simulink library "wt_blockset_v3"  (Simulink 6.0)
settings: Solver=ode45  SolverMode=SingleTasking  StartTime=0.0  StopTime=10.0  RelTol=1e-3
undefined symbols (not defined in the file): f1, get, j, Kmode, Type, u0
libraries: simulink_extras x12, simulink3 x5, simulink x4, dspinverses x1, dspmtrx3 x1, dspsnks4 x1
(part 1 of 7)
Description:
  | Currently the toolbox can run under Release 7.0.0 (Service Pack 1).
  | Since there are major differences between this Matlab Release and the
  | previous ones, it is highly recommended to use the Toolbox just with
  | Release 7.0.0 or higher.
  | 
  | Many thanks for feedbacks and improvements in particular to:
  | - my colleagues from Risø: Anca Hansen, Poul Sørensen, Nic Cutululis
  | - James F. Conroy
  | - Gabrielle Gail
  | 
  | Also, many thanks to all the users.
  | 
  | Florin
settings Model: Creator=Florin iov  LastModifiedBy=fi  ModifiedComment=fi -- Thu Jun 08 10:02:30 2006 -- Version 3.0.19
settings Model: ModifiedHistory=|
  | fi -- Thu Jun 08 10:02:30 2006 -- Version 3.0.19
  | 
  | 
  | fi -- Tue Oct 25 13:03:19 2005 -- Version 3.0.18
  | 
  | 
  | fi -- Tue Oct 25 13:01:51 2005 -- Version 3.0.17
  | 
  | 
  | fi -- Tue Oct 25 13:01:21 2005 -- Version 3.0.16
  | 
  | 
  | fi -- Tue Oct 25 12:57:57 2005 -- Version 3.0.15
  | 
  | 
  | fi -- Tue Oct 25 12:21:51 2005 -- Version 3.0.14
  | 
  | 
  | fi -- Tue Oct 25 12:15:48 2005 -- Version 3.0.13
  | 
  | 
  | fi -- Tue Oct 25 12:00:01 2005 -- Version 3.0.12
  | Updates: Grid Model, Line Model, Wind Model SB, Capacitor Bank Model, Discrete PLL and PI Controller
  | 
  | fi -- Mon Oct 24 09:19:02 2005 -- Version 3.0.11
  | 
  | 
  | fi -- Thu Jun 02 08:52:48 2005 -- Version 3.0.10
  | 
  | 
  | fi -- Thu Jun 02 08:43:54 2005 -- Version 3.0.9
  | 
  | 
  | fi -- Thu Jun 02 08:40:14 2005 -- Version 3.0.8
  | 
  | 
  | fi -- Wed May 25 13:16:38 2005 -- Version 3.0.7
  | 
  | 
  | fi -- Wed May 25 13:08:05 2005 -- Version 3.0.6
  | 
  | 
  | fi -- Wed May 25 11:45:18 2005 -- Version 3.0.5
  | 
  | 
  | fi -- Wed May 25 11:38:20 2005 -- Version 3.0.3
  | 
  | 
  | fi -- Wed May 25 11:38:20 2005 -- Version 3.0.3
  | 
  | 
  | fi -- Wed May 25 11:25:12 2005 -- Version 3.0.2
settings OptimizationCC: BooleanDataType=off
settings DebuggingCC: SolverPrmCheckMsg=none
settings HardwareCC: TargetUnknown=on

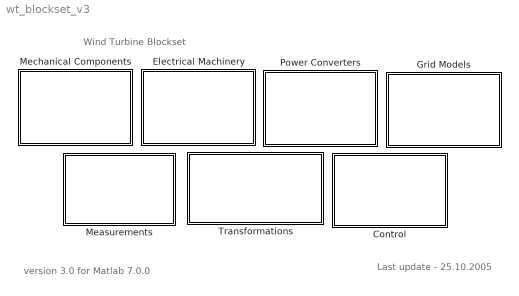
== system wt_blockset_v3 ==
  note: Wind Turbine Blockset
  note: Last update - 25.10.2005
  note: version 3.0 for Matlab 7.0.0
  Control : Subsystem
      mask Display: disp('Control')
  Electrical Machinery : Subsystem
      mask Display: disp('Electrical\nMachinery')
  Grid Models : Subsystem
      mask Display: disp('Grid\nModels')
  Measurements : Subsystem
      mask Display: disp('Measurements')
  Mechanical Components : Subsystem
      mask Display: disp('Mechanical\nComponents')
  Power Converters : Subsystem
      mask Display: disp('Power\nConverters')
  Transformations : Subsystem
      mask Display: disp('Transformations')

== system wt_blockset_v3/Control ==
  note: Control Blocks
  "Active Stall Controller " : Subsystem  mask{K=0.01, Ti=0.0025, ka=500, Kpitch=1000, P=300, avg_wind=11.5, rated_wind=11.8}
      mask prompts: K "Gain Power Controller"; Ti "Integration time constant Power Controller"; ka "Gain anti wind-up Power Controller"; Kpitch "Gain Pitch Controller"; P "Allowed Overpower [kW]"; avg_wind "Average Wind Speed [m/sec]"; rated_wind "Rated Wind Speed"
      mask init:
      | Pallowed=P;
      mask Display: disp('Active\nStall\nController')
  Control P&Q  2 MW DFIG : Subsystem  mask(Control P & Q for double feed induction generator){param=[0.0011, 7e-5, 0.0013, 7.5e-5, 2.9936e-3], p=2, fs=50}
      mask prompts: param "Electrical parameters [Rs Lsgm_s Rr Lsgm_r Lm]"; p "Number of pole pais"; fs "Base frequency [Hz]"
      mask help: Control of active and reactive power in synchronous reference frame for DFIG.
      mask init:
      | Rs=param(1); Lsgm_s=param(2); Rr=param(3); Lsgm_r=param(4);
      | Lm=param(5); Lss=Lsgm_s+Lm; Lrr=Lsgm_r+Lm; D=Lss*Lrr-Lm^2;
      | T=D/Lss; Tpr=(Lm^2)/Lss;
      | tau_1=T/Rr;  tau_2=Rr;
      mask Display: disp('Control\nP&Q')
  PI Controller anti wind-up : Subsystem  mask{K=0.09, Ti=0.016, ka=10, maxim=1000, init_cond=2}
      mask prompts: K "Proportional Constant"; Ti "Integrate constant"; maxim "Limits"; init_cond "initial"
      mask Display: disp('PI')
  WT Controller 2 MW DFIG : Subsystem  mask(Wind Turbine Controller){Kp_power=400, Ti_power=1, Kp_speed=0.02, Ti_speed=10}
      mask prompts: Kp_power "Gain Power Controller"; Ti_power "Integration Time Power Controller"; Kp_speed "Gain Speed Controller"; Ti_speed "Integration Time Speed Controller"
      mask help:
      | Implements the wind turbine controller for a 2MW DFIG WT.
      | Power input is in per unit from the total deliver power.
  control soft starter : Subsystem  TreatAsAtomicUnit=on
      mask Type: Firing angle control for soft starter
      mask Description: Implements the control for soft starter
      mask Display: disp('   ')
  discrete PI Controller anti windup : Subsystem  mask{Kp=2, Ti=0.5, Ka=0, OutLim=1, Ts=1e-2, InitCond=0}
      mask prompts: Kp "Gain"; Ti "Integration Time Constant"; Ka "gain antiwindup"; OutLim "Output limit"; Ts "Sampling time"; InitCond "Initial condition"
      mask Display: disp('Discrete PI')

== system wt_blockset_v3/Electrical Machinery ==
  note: Electrical Machinery Library
  C S-Function based  Models : Subsystem
      mask Display: disp('C S-Function\nbased  Models')
  Simulink Blocks  based Models : Subsystem
      mask Display: disp('Simulink Blocks\n based Models')

== system wt_blockset_v3/Grid Models ==
  note: Sources
  note: Cables & Distribution Lines
  note: others
  note: Transformers
  3-ph line 1 : Subsystem  mask(3-phase distribution line){d=3.3, R=0.115, L=0.19/314, C=0.52e-6}
      mask prompts: d "Line length [km]"; R "Line resistance [ohms/km]"; L "Line inductance [H/km]"; C "Line capacitance [F/km]"
      mask init:
      | Zc=sqrt(L/C);
      | tdelay=d*sqrt(L*C);
      | atten=exp(-(R/2)*d*sqrt(C/L));
      | buffer_size=20000;
  3-ph line 2 : Subsystem  mask(3-phase distribution line){d=4, R=0.115, L=0.2/314, C=0.1e-6}
      mask prompts: d "Line length [km]"; R "Line resistance [ohms/km]"; L "Line inductance [H/km]"; C "Line capacitance [F/km]"
      mask init:
      | Zc=sqrt(L/C);
      | tdelay=d*sqrt(L*C);
      | atten=exp(-(R/2)*d*sqrt(C/L));
      | buffer_size=20000;
  3-phase 3 limb  C S-Function : Subsystem  mask(ABC/abc Dynamic Model of 3-phase 3 limb transformer){power=[2e6 3489], voltage=[31500 690/sqrt(3)], frequency=50, hv_winding=[4.5565 51.227], lv_winding=[2.93 51.227], core_ratio=0.33}
      mask prompts: power "Rated power, No-load losses [Sr (VA), Po (W)]"; voltage "Rated phase voltages [U1r (V), U2r (V)]]"; frequency "Rated frequency [Hz]"; hv_winding "High-voltage windings [Rhv  X_hv] [ohms]"; lv_winding "Low-voltage windings [Rlv X_lv] [ohms]"; core_ratio "Core ratio (l/L)"
      mask help:
      | Implements a dynamic model of a 3-phase 2-windings transformer in natural frame (ABC/abc). Core geometry is taken into account.
      | Connection Type Dyn1.
      mask init:
      | %%%%%%%%%%%%%%%%%%%%%%%%%%%%%%%%%%%%%%%%%%%%%%%%%%%%%%%%%
      | % Coefficients for ABC/abc Model of 3-phase Transformer %
      | %           Core structure is taken into account        %
      | %               Last Update 6.08.2002                   %
      | %%%%%%%%%%%%%%%%%%%%%%%%%%%%%%%%%%%%%%%%%%%%%%%%%%%%%%%%%
      | 
      | %Base power
      | Sbase=power(1);
      | 
      | %No load losses
      | Po=power(2);
      | 
      | %Base HV voltage
      | Ubase_hv=voltage(1);
      | 
      | %Base HV voltage
      | Ubase_lv=voltage(2);
      | 
      | %Base impedance LV
      | Zbase_lv=3*(Ubase_lv^2)/Sbase;
      | 
      | %Transformer turns ratio
      | alpha_T=Ubase_hv/Ubase_lv;
      | 
      | %No load losses per unit
      | Po_pu=Po/Sbase;
      | 
      | %
      | omg=2*pi*frequency;
      | 
      | %High-voltage windings
      | R1=hv_winding(1);
      | X1=hv_winding(2);
      | 
      | %Low-voltage windings
      | R2=lv_winding(1);
      | X2=lv_winding(2);
      | 
      | %%%%%%%%%%%%%%%%%%%%%%%%%%%%%%%%%%%%%%%%%%%%%%%%%%%%%%%%%%%%%
      | 
      | Lsgm=[ X1,     0,     0,     0,     0,     0;...
      |         0,    X1,     0,     0,     0,     0;...
      |         0,     0,    X1,     0,     0,     0;...
      |         0,     0,     0,    X2,     0,     0;...
      |         0,     0,     0,     0,    X2,     0;...
      |         0,     0,     0,     0,     0,    X2]./omg;
      | 
      | 
      | R=[    R1,     0,     0,     0,     0,     0;...
      |         0,    R1,     0,     0,     0,     0;...
      |         0,     0,    R1,     0,     0,     0;...
      |         0,     0,     0,    R2,     0,     0;...
      |         0,     0,     0,     0,    R2,     0;...
      |         0,     0,     0,     0,     0,    R2];
      | 
      | a=core_ratio;
      | 
      | %3limb core
      | %Ideal transformer matrix
      | 
      | k1=-0.5*(1+2*a)/(1+a);
      | k2=-0.5/(1+a);
      | k3=(1+2*a)/(1+a);
      | 
      | Ti=[  1, k1, k2,  1, k1, k2;...
      |      k1, k3, k1, k1, k3, k1;...
      |      k2, k1,  1, k2, k1,  1;...
      |       1, k1, k2,  1, k1, k2;...
      |      k1, k3, k1, k1, k3, k1;...
      |      k2, k1,  1, k2, k1,  1];
      | 
      | T=Ti(1:3,1:3);
      | 
      | dlt=0.001*eye(3,3);
      | 
      | Z=j*(dlt+T);
      | 
      | U=[exp(j*0);exp(-j*2*pi/3);exp(+j*2*pi/3)];
      | 
      | I=Z\U;
      | 
      | Iu=mean(abs(I));
      | 
      | Io_pu=0.002;
      | 
      | PU=real(I'*T*(I));
      | 
      | zeta=Iu/Io_pu;
      | 
      | c=zeta^2*Po_pu/PU;
      | 
      | k=sqrt((zeta^2-c^2)/omg^2);
      | 
      | R0=c*Zbase_lv*alpha_T^2*Ti;
      | L0=k*Zbase_lv*alpha_T^2*Ti;
      | 
      | Re=R+R0;
      | Le=Lsgm+L0;
      | 
      | a=-Le\Re;
      | 
      | b=inv(Le);
      | 
      | init_cond = [0 0 0 0 0 0];
      mask Display: disp('3phase 3 limb\n Transformer')
  3-phase 3 limb  Transformer : Subsystem  mask(ABC/abc Dynamic Model of 3-phase 3 limb transformer){power=[2e6 3489], voltage=[31500 690/sqrt(3)], frequency=50, hv_winding=[4.5565 51.227], lv_winding=[2.93 51.227], core_ratio=0.33}
      mask prompts: power "Rated power, No-load losses [Sr (VA), Po (W)]"; voltage "Rated phase voltages [U1r (V), U2r (V)]]"; frequency "Rated frequency [Hz]"; hv_winding "High-voltage windings [Rhv  X_hv] [ohms]"; lv_winding "Low-voltage windings [Rlv X_lv] [ohms]"; core_ratio "Core ratio (l/L)"
      mask help:
      | Implements a dynamic model of a 3-phase 2-windings transformer in natural frame (ABC/abc). Core geometry is taken into account.
      | Connection Type Dyn1.
      mask init:
      | %%%%%%%%%%%%%%%%%%%%%%%%%%%%%%%%%%%%%%%%%%%%%%%%%%%%%%%%%
      | % Coefficients for ABC/abc Model of 3-phase Transformer %
      | %           Core structure is taken into account        %
      | %               Last Update 6.08.2002                   %
      | %%%%%%%%%%%%%%%%%%%%%%%%%%%%%%%%%%%%%%%%%%%%%%%%%%%%%%%%%
      | 
      | %Base power
      | Sbase=power(1);
      | 
      | %No load losses
      | Po=power(2);
      | 
      | %Base HV voltage
      | Ubase_hv=voltage(1);
      | 
      | %Base HV voltage
      | Ubase_lv=voltage(2);
      | 
      | %Base impedance LV
      | Zbase_lv=3*(Ubase_lv^2)/Sbase;
      | 
      | %Transformer turns ratio
      | alpha_T=Ubase_hv/Ubase_lv;
      | 
      | %No load losses per unit
      | Po_pu=Po/Sbase;
      | 
      | %
      | omg=2*pi*frequency;
      | 
      | %High-voltage windings
      | R1=hv_winding(1);
      | X1=hv_winding(2);
      | 
      | %Low-voltage windings
      | R2=lv_winding(1);
      | X2=lv_winding(2);
      | 
      | %%%%%%%%%%%%%%%%%%%%%%%%%%%%%%%%%%%%%%%%%%%%%%%%%%%%%%%%%%%%%
      | 
      | Lsgm=[ X1,     0,     0,     0,     0,     0;...
      |         0,    X1,     0,     0,     0,     0;...
      |         0,     0,    X1,     0,     0,     0;...
      |         0,     0,     0,    X2,     0,     0;...
      |         0,     0,     0,     0,    X2,     0;...
      |         0,     0,     0,     0,     0,    X2]./omg;
      | 
      | 
      | R=[    R1,     0,     0,     0,     0,     0;...
      |         0,    R1,     0,     0,     0,     0;...
      |         0,     0,    R1,     0,     0,     0;...
      |         0,     0,     0,    R2,     0,     0;...
      |         0,     0,     0,     0,    R2,     0;...
      |         0,     0,     0,     0,     0,    R2];
      | 
      | a=core_ratio;
      | 
      | %3limb core
      | %Ideal transformer matrix
      | 
      | k1=-0.5*(1+2*a)/(1+a);
      | k2=-0.5/(1+a);
      | k3=(1+2*a)/(1+a);
      | 
      | Ti=[  1, k1, k2,  1, k1, k2;...
      |      k1, k3, k1, k1, k3, k1;...
      |      k2, k1,  1, k2, k1,  1;...
      |       1, k1, k2,  1, k1, k2;...
      |      k1, k3, k1, k1, k3, k1;...
      |      k2, k1,  1, k2, k1,  1];
      | 
      | T=Ti(1:3,1:3);
      | 
      | dlt=0.001*eye(3,3);
      | 
      | Z=j*(dlt+T);
      | 
      | U=[exp(j*0);exp(-j*2*pi/3);exp(+j*2*pi/3)];
      | 
      | I=Z\U;
      | 
      | Iu=mean(abs(I));
      | 
      | Io_pu=0.002;
      | 
      | PU=real(I'*T*(I));
      | 
      | zeta=Iu/Io_pu;
      | 
      | c=zeta^2*Po_pu/PU;
      | 
      | k=sqrt((zeta^2-c^2)/omg^2);
      | 
      | R0=c*Zbase_lv*alpha_T^2*Ti;
      | L0=k*Zbase_lv*alpha_T^2*Ti;
      | 
      | Re=R+R0;
      | Le=Lsgm+L0;
      | 
      | a=-Le\Re;
      | 
      | b=inv(Le);
      mask Display: disp('3phase 3 limb\n Transformer')
  3-phase source : Subsystem  mask(3 - Phase Voltage Source){Uf=220, fs=50}
      mask prompts: Uf "Phase voltage [V]"; fs "Fundamental frequency [Hz]"
  Capacitor Bank RC : Subsystem  mask(Capacitor Bank RC){R=1, CmF=21.737}
      mask prompts: R "Series rezistor [ohms]"; CmF "Branch Capacitor [mF]"
      mask init:
      | C=CmF*1e-3;
      mask Display: disp('Capacitor\nBank')
  Capacitor Bank RC modified : Subsystem  mask(Capacitor Bank RC){P=25, Q=500, Vl=0.69}
      mask prompts: P "Dissipated Real Power [W]"; Q "Rated Reactive Power [kVAr]"; Vl "Rated Line Voltage [kV]"
      mask init:
      | Vl = Vl*1e3 ;
      | Q = Q*1e3 ;
      | f = 50 ;
      | omega = 2*pi*f ;
      | 
      | % -------------------------------------------------------------------------
      | 
      | 
      | % Now evaluate the first guess, which is important in Newton-Raphson
      | % algorithms.
      | 
      | % Since the resistance is parasitic in an a real capacitor, R=0 is a decent first guess
      | R = 0 ;
      | % The first guess value for C is the formula for an ideal capacitor
      | C = Q/(Vl^2*omega) ;
      | 
      | % The iterated values for R and C need to be initially at values that are quite different from the first guess values
      | R_prev = 1000 ;
      | C_prev = 1000 ;
      | 
      | % The iteration formula is as follows
      | % -------------------------------------------
      | 
      | %    | a11 a12 |   | dR |     | f(R,C) |
      | %    |         | . |    | = - |        |
      | %    | a21 a22 |   | dC |     | g(R,C) |
      | 
      | %    R(n+1) = R(n) + dR
      | %    C(n+1) = C(n) + dC
      | 
      | %---------------------------------------------
      | 
      | 
      | i = 0 ; % The number of iterations
      | 
      | while((abs(R-R_prev)>0.00000001)|(abs(C-C_prev)>0.00000001))
      |     
      |     R_prev = R ; % Update the previous guess for R
      |     C_prev = C ; % Update the previous guess for C
      |     
      |     % Evaluate the two non-linear functions
      |     f = P*(R^2)+(P/((omega*C)^2))-(Vl^2*R) ;
      |     g = (Q*omega*C*R^2)+(Q/(omega*C))-Vl^2 ;
      | 
      |     % Now get the factors that you require
      |     a11 = P*2*R - Vl^2 ;
      |     a12 = -2*P/(omega^2*C^3) ;
      |     a21 = Q*2*R ;
      |     a22 = (-Q*2/(omega^2*C^3))-(Vl^2/omega^2)-(1/(C^2)) ; 
      | 
      |     A = [a11 a12;a21 a22] ;
      | 
      |     b = [f;g] ;
      | 
      |     y = -(A\b) ; % The MATLAB convention for solving by Gaussian Elimination
      |     
      |     R = R_prev+y(1) ; % Update the guess for R
      |     C = C_prev+y(2) ; % Update the guess for C
      |     
      |     % This loop performs iteration control!!
      |     i = i+1 ;
      |     if i==500000
      |         break ;
      | 	end
      | end
      | R;
      | C;
      mask Display: disp('Capacitor\nBank')
  Capacitor Bank RLC : Subsystem  mask(Capacitor Bank RLC){R=0.0001, X=0.00034, CmF=0.0005}
      mask prompts: R "Series rezistor [ohms]"; X "Reactor [ohms]"; CmF "Capacitance [mF]"
      mask init:
      | L=X/(2*pi*50);
      | C=CmF*1e-3;
      mask Display: disp('Capacitor\nBank')
  Circuit breaker : Subsystem  mask{to=1/50, Ro=100, tc=1/50, Rc=100}
      mask prompts: to "Opening time"; Ro "Opening resistance"; tc "Closing time"; Rc "Closing resistance"
  DC-link circuit : Subsystem  mask(DC-link circuit){R=0.001, CuF=21.737, init_cond=0}
      mask prompts: R "Series rezistor [ohms]"; CuF "Capacitor [uF]"; init_cond "Initial DC-link Voltage [V]"
      mask init:
      | C=CuF*1e-6;
      mask Display: disp('DC\nLink')
  GRID 1 : Subsystem  mask(3 - Phase Voltage Source){Uf=31500, R=0, X=1.5, fs=50}
      mask prompts: Uf "Phase voltage [V]"; R "Resistance"; X "Reactance"; fs "Fundamental frequency [Hz]"
  GRID 2 : Subsystem  mask{fg=50, Vpcc=30000, Ssc=20, phi_grid=80, Rf=0.31, SCR=5, tsc=0.3, td=0.5}
      mask prompts: fg "fgrid [Hz]"; Vpcc "Vpcc line-line  rms [V]"; Ssc "Short-circuit Power (MVA)"; phi_grid "Grid angle [degrees]"; Rf "Short-circuit resistance"; SCR "Short-circuit ratio x/r"; tsc "Short-circuit occurance"; td "Short-circuit duration"
      mask init:
      | V1=Vpcc/sqrt(3);
      | 
      | tg_alpha=tan(phi_grid*pi/180);
      | Zsc=Vpcc^2/(Ssc*1e6);
      | 
      | R=sqrt(Zsc^2/(1+tg_alpha^2));
      | X=R*tg_alpha;
      | L=X/(2*pi*50);
      | 
      | %Short-circuit inductance
      | Lf=SCR*Rf/(2*pi*50);
  Harmonic Voltage Source : Subsystem  mask(Harmonic Voltage Source){phase_o=178.2, h3=on, h5=on, h7=on, h9=on, h11=on, h13=on}
      mask prompts: phase_o "Initial phase [deg]"; h3 "Insertion of 3rd harmonic"; h5 "Insertion of 5th harmonic"; h7 "Insertion of 7th harmonic"; h9 "Insertion of 9th harmonic"; h11 "Insertion of 11th harmonic"; h13 "Insertion of 13th harmonic"
      mask help: Implements a harmonic voltage source according with Standard EN61000-2-2.
      mask init:
      | gama_0=phase_o*pi/180;
  Voltage  source complex : Subsystem  mask(3 - Phase Voltage Source){Uf=960}
      mask prompts: Uf "Phase voltage [V]"

== system wt_blockset_v3/Measurements ==
  note: Measurements
  Discrete PLL : Subsystem  mask(Discrete PLL){Kp=92, Ti=0.1739, Ka=10, limit=500, Vrms=230, fgrid=50, ffilter=10, Ts=1/5000, init_cond=[0 0 0 230]}
      mask prompts: Kp "Gain Controller"; Ti "Integration Time Controller"; Ka "Gain Antiwindup Controller"; limit "Limit Output Controller"; Vrms "RMS Voltage"; fgrid "Fundamental frequency"; ffilter "Filter cut-off frequency"; Ts "Sampling Time"; init_cond "Initial Condition Integrators"
      mask help: implements a discrete Phase Locked Loop.
      mask Display: disp('Discrete PLL')
  Moving Average Filter : Subsystem  mask(Moving Average Filter){Tav=60, init=10}
      mask prompts: Tav "Averaging time interval [sec]"; init "Initial condition"
      mask help: Implements a Moving average filter in time domain
      mask Display: disp('Moving\nAverage')
  P & Q dq : Subsystem
      mask Type: P & Q 1st approach
      mask Description: Calculate active and reactive power based on dq components
      mask Display: disp('P&Q')
  P & Q mono phase : Subsystem  mask(Active & Reactive Power ){f=50}
      mask prompts: f "Fundamental frequency (Hz):"
      mask Display: disp('P&Q\n 1 phase')
  P & Q three phase : Subsystem  mask(Active & Reactive Power ){f=50}
      mask prompts: f "Fundamental frequency (Hz):"
      mask Display: disp('P&Q\n 3-phase')
  Period : Subsystem
      mask Type: Period calculator
      mask Description: Find period for a sinusoidal signals.
      mask Display: disp('')
  Phase Locked Loop : Subsystem  mask(Phase Locked Loop){fs=50, Kp=180.03, Ti=0.00786}
      mask prompts: fs "Fundamental frequency (Hz):"; Kp "Proportional coefficient"; Ti "Integration time constant [sec]"
      mask help: Implements a Phase Locked Loop for grid angle detection
      mask Display: disp('PLL')
  S complex : Subsystem
      mask Type: P & Q
      mask Description: Calculate active and reactive power based on complex inputs
      mask Display: disp('S')
  average wind : Subsystem  mask(Computes the average value of the wind on a given interval){T_period=60, T_sample=0.05}
      mask prompts: T_period "Time period [sec]"; T_sample "Sample time [sec]"
      mask init:
      | N_samples=T_period/T_sample;
      mask Display: disp('Average\nwind')
  power spectra : Subsystem  mask(power spectra){t_sample=0.05}
      mask prompts: t_sample "Sample period"

== system wt_blockset_v3/Mechanical Components ==
  note: Wind Models
  note: Gearbox Models
  note: Rotor Models
  One-mass model : Subsystem  mask{J=90}
      mask prompts: J "Moment of inertia [Nm2]"
      mask Display: disp('E M')
  One-mass model with gear-box : Subsystem  mask(Simple Gearbox){Jem=90, Jwt=49.5e5, K=83.531, init_speed=1.87355}
      mask prompts: Jem "Electric machinery - Moment of inertia [kg m2]"; Jwt "Wind turbine rotor - Moment of inertia [kg*m2]"; K "Gearbox ratio"; init_speed "Initial condition [omg_wt (rad/sec)]"
      mask init:
      | J=Jem*K^2+Jwt;
      mask Display: disp('E M\nGear box')
  Two-mass model : Subsystem  TreatAsAtomicUnit=on  mask(Gearbox with torsional torque){Jem=90, Jwt=49.5e5, Kshaft=114e6, Dshaft=755.658e3, Kgear=83.531, init=[156.5 1.87355]}
      mask prompts: Jem "Electric machine - Moment of inertia:  Jem [ kg*m2]"; Jwt "Wind turbine rotor - Moment of inertia:  Jwt [kg*m2]"; Kshaft "Shaft stiffness:  Kshaft [ Nm/rad]"; Dshaft "Damping coeficient of shaft:  Dshaft [Nm sec/rad]"; Kgear "Gearbox ratio"; init "Initial conditions [omg_em (rad/sec), omg_wt (rad/sec) ]"
      mask help: Implements a gearbox with torsional torque.
      mask Display: disp('Drive Train')
  Two-mass model 'C' S-Function : Subsystem  TreatAsAtomicUnit=on  mask(Gear box with torsional torques){Jem=90, Jwt=49.5e5, Kshaft=114e6, Dshaft=755.658e3, Kgear=83.531, init_cond=[156.5 0 1.87355 0]}
      mask prompts: Jem "Electric machine - Moment of inertia:  Jem [ kg*m2]"; Jwt "Wind turbine rotor - Moment of inertia:  Jwt [kg*m2]"; Kshaft "Shaft stiffness:  Kshaft [ Nm/rad]"; Dshaft "Damping coeficient of shaft:  Dshaft [Nm sec/rad]"; Kgear "Gearbox ratio"; init_cond "Initial conditions [omg_em(rad/s) th_em(rad) omg_wtr(rad/s) th_wtr(rad)]"
      mask help:
      | Implemets the dynamic model of a gearbox with torsional torques.
      | Equations are written at the low speed shaft (wind turbine side).
      mask Display: disp('Drive Train')
  Wind Model SB-1 : Subsystem  TreatAsAtomicUnit=on  mask(Wind Model using Simulink Band-limited white noise generator){D_rotor=72, v_mean=10, roughness=600, turb_int=12, T_sample=0.05}
      mask prompts: D_rotor "Rotor diameter [m]"; v_mean "Average wind speed [m/sec]"; roughness "Length scale [m]"; turb_int "Turbulence intensity [%]"; T_sample "Sample time [sec]"
      mask help:
      | Implements a rotor wind model developped by RISOE National Laboratory based on Kaimal spectra. The model takes into account the rotational turbulences and the tower shadow.
      | This model uses the built-in band-limited white noise generator from Simulink with different seeds.
      mask init:
      | r = D_rotor/2;
      | sigma = v_mean*turb_int/100;
      | var = sigma^2;
      | c = roughness/(2*pi*v_mean);
      | d = r/v_mean;
      | trans=sigma*sqrt(roughness/v_mean);
      | random=[256, 894, 31];
      mask Display: disp('Wind\nModel\n(SB-1)')
  Wind Model SB-2 : Subsystem  TreatAsAtomicUnit=on  mask(Wind Model using Simulink Band-limited white noise generator){D_rotor=72, L=600, turb_int=12, T_sample=0.05}
      mask prompts: D_rotor "Rotor diameter [m]"; L "Length scale [m]"; turb_int "Turbulence intensity [%]"; T_sample "Sample time [sec]"
      mask help:
      | Implements a rotor wind model developped by RISOE National Laboratory based on Kaimal spectra. The model takes into account the rotational turbulences and the tower shadow.
      | This model uses the built-in band-limited white noise generator from Simulink
      mask init:
      | r = D_rotor/2;
      | random=[256, 894, 31];
      mask Display: disp('Wind\nModel\n(SB-2)')
  Wind Model ZA-1 : Subsystem  TreatAsAtomicUnit=on  mask(Wind Model using Marsaglia's Ziggurat Algorithm){D_rotor=72, v_mean=10, roughness=600, turb_int=12, T_sample=0.05}
      mask prompts: D_rotor "Rotor diameter [m]"; v_mean "Average wind speed [m/sec]"; roughness "Length scale [m]"; turb_int "Turbulence intensity [%]"; T_sample "Sample time [sec]"
      mask help:
      | Implements a rotor wind model developped by RISOE National Laboratory based on Kaimal spectra. The model takes into account the rotational turbulences and the tower shadow.
      | The white noise generators uses a new block based on a 'C' S-Function which implements the Marsaglia's Ziggurat Algorithm.
      mask init:
      | r = D_rotor/2;
      | sigma = v_mean*turb_int/100;
      | var = sigma^2;
      | c = roughness/(2*pi*v_mean);
      | d = r/v_mean;
      | trans=sigma*sqrt(roughness/v_mean);
      mask Display: disp('Wind\nModel\n(ZA-1)')
  Wind Model ZA-2 : Subsystem  TreatAsAtomicUnit=on  mask(Wind Model using Marsaglia's Ziggurat Algorithm){D_rotor=72, L=600, turb_int=12, T_sample=0.05}
      mask prompts: D_rotor "Rotor diameter [m]"; L "Length scale [m]"; turb_int "Turbulence intensity [%]"; T_sample "Sample time [sec]"
      mask help:
      | Implements a rotor wind model developped by RISOE National Laboratory based on Kaimal spectra. The model takes into account the rotational turbulences and the tower shadow.
      | The white noise generators uses a new block based on a 'C' S-Function which implements the Marsaglia's Ziggurat Algorithm.
      mask init:
      | r = D_rotor/2;
      mask Display: disp('Wind\nModel\n(ZA-2)')
  Wind Turbine Rotor Active Stall : Subsystem  mask(Aerodynamic model for wind turbine){R=40, ro_air=1.25, cut_in=3, cut_out=25, Tact=0}
      mask prompts: R "Blade radius [m]"; ro_air "Air density [kg m3]"; cut_in "Cut in speed [m/sec]"; cut_out "Cut out speed [m/sec]"; Tact "Time constant for pitch actuator [sec]"
      mask init:
      | load cp_cq;
      | Ctorque=cq(2:5:102,2:5:182);
      | clear Cp cq
      mask Display: plot(20,0,120,200,[45,35,35,45,75,75,45],[85,92,108,115,115,85,85],[55,50,70,65],[115,180,190,115],[55,50,70,65],[85,10,20,85],[75,85],[102,102],[75,85],[98,98],[105,85,85,105],[80,85,115,120])
  Wind Turbine Rotor Variable Pitch : Subsystem  mask(Aerodynamic model for wind turbine){R=40, ro_air=1.25, cut_in=3, cut_out=25, Tact=0}
      mask prompts: R "Blade radius [m]"; ro_air "Air density [kg m3]"; cut_in "Cut in speed [m/sec]"; cut_out "Cut out speed [m/sec]"; Tact "Time constant for pitch actuator [sec]"
      mask init:
      | load cp_cq;
      | Ctorque=cq(2:5:102,2:5:182);
      | clear Cp cq
      mask Display: plot(20,0,120,200,[45,35,35,45,75,75,45],[85,92,108,115,115,85,85],[55,50,70,65],[115,180,190,115],[55,50,70,65],[85,10,20,85],[75,85],[102,102],[75,85],[98,98],[105,85,85,105],[80,85,115,120])

== system wt_blockset_v3/Power Converters ==
  note: Power Converters Models
  note: Power Converters RMS Models
  note: Modulation Strategies
  3-phase Diode Bridge Rectifier : Subsystem
      mask Type: 3 phase Diode Bridge Rectifier
      mask Description: Implements a model for 3 phase Diode Bridge Rectifier.
      mask Display: disp('')
  Average PWM Strategy : Subsystem  mask(Average sinusoidal PWM Strategy with Simulink Blocks){third=on}
      mask prompts: third "Insertion of third harmonic"
      mask help: Implements an average model of a sinusoidal PWM strategy using Simulink Blocks.
      mask Display: disp('Average\nPWM')
  Average SVM Strategy : Subsystem
      mask Type: Average SVM Strategy with Simulink Blocks
      mask Description: Implements an average model of a SV-PWM strategy using Simulink Blocks.
      mask Display: disp('Average\nSVM')
  Average SVM Strategy C_Sfun : Subsystem
      mask Type: Average SVM Strategy C-SFun
      mask Description: Implements an average model of a SV-PWM strategy using a C-SFunction.
      mask Display: disp('Average\nSVM')
  RMS - Soft Starter : Subsystem  mask(RMS Model for Soft Starter){}
      mask help: Implements an RMS model for soft-starter based on a look-up table for extincton angle of the SCR.
      mask init:
      | ext_angle_ss%%%%%%%%%%%%%%%%%%%%%%%%%%%%%%%%%%%%%%%%%%%
      | % Extinction angle tabel for Soft Starter %
      | %       Last Update 10.05.2002            %
      | %%%%%%%%%%%%%%%%%%%%%%%%%%%%%%%%%%%%%%%%%%%
      | 
      | ext_angle=[ 180  180   180  180   180   180   180   180   180   180   180   180   180;...
      |             195  195   195  195   195   195   194.9 194.8 194.6 193.9 192.4 189   180;...
      |             210  210   210  209.9 209.7 209.3 208.6 207.5 205.7 202.9 198.5 191.5 180;...
      |             225  225   225  225   224.2 222.8 220.9 218.1 214.3 209.1 202.1 192.8 180;...
      |             240  240   240  240   240   237.1 233.2 228.2 221.9 214.2 204.9 193.6 180;...
      |             255  255   255  255   255   255   247.9 239.5 230   219.3 207.4 194.3 180;...
      |             270  270   270  270   270   270   270   255   240   225   210   195   180];
  SVM Strategy : Subsystem  mask(SVM-Strategy){fs=1000, Udc=600, td=3.2e-6, mpw=5.6e-6, mct=.4e-6*10, dp=0}
      mask prompts: fs "Parameters:Switching sampling frequency 'fs' [Hz] :"; Udc "DC Link voltage 'Udc' [V] :"; td "Inverter Deadtime 'td' [sec] :"; mpw "Minimum Puls-Width 'mpw' [sec] :"; mct "CPU cycle time 'cmt' [sec] :"; dp "Pulse-Dropping : 0-disabled, 1-enabled"
      mask help: SPACE VECTOR MODULATION - based PWM VSC
      mask Display: plot(0,0,100,100,[3,5,5,10,10,15,15,25,25,30,30,40,40,45,45,50,50,55,55,60,60,70,70,75,75,85,85,90,90,95,95,97],[50,50,10,10,50,50,10,10,50,50,10,10,50,50,10,10,90,90,50,50,90,90,50,50,90,90,50,50,90,90,50,50],[2,98],[50,50])
  Sinus PWM : Subsystem  mask(Sinus PWM Strategy){mf=15, f1=50}
      mask prompts: mf "Amplitude modulation index"; f1 "Fundamental frequency"
  Soft-Starter : Subsystem  mask(Soft Starter){ConType=Delta, fs=50, init=[0 1 1]}
      mask prompts: ConType "Connection Type"; fs "Fundamental frequency [Hz]"; init "Initial states"
      mask help: Implements a Soft-Starter model for star, delta and branch-delta connection using switching functions.
      mask init:
      | init_a=init(1);
      | init_b=init(2);
      | init_c=init(3);
      mask StyleString: popup(Star|Delta|Branch Delta),edit,edit
  Switching PWM Strategy : Subsystem  mask(Switching sinusoidal PWM with Simulink Blocks){carrier=1000, dead_time=3.2e-6, min_pw=5e-6, dp=on, third=on}
      mask prompts: carrier "Carrier frequency [Hz]"; dead_time "Dead time [sec]"; min_pw "Minimum pulse width [sec]"; dp "Pulse dropping"; third "Insertion of third harmonic"
      mask help: Implements a switching model of a sinusoidal PWM strategy using Simulink Blocks.
      mask init:
      | mpw=0.5*min_pw;
      mask Display: disp('Switching\nPWM')
  Switching SVM Strategy : Subsystem  mask(Switching SVM Strategy with Simulink Blocks){fsw=4000, dead_time=3.2e-6, min_pw=5e-6, dp=off}
      mask prompts: fsw "Switching frequency"; dead_time "Dead time [sec]"; min_pw "Minimum pulse width [sec]"; dp "Pulse dropping"
      mask help: Implements a switching model of a SV-PWM strategy using Simulink Blocks.
      mask init:
      | Tsw=1/fsw;
      | mpw=0.5*min_pw;
      mask Display: disp('Switching\nSVM')
  Switching SVM Strategy C_Sfun : Subsystem  mask(Switching SVM Strategy){fsw=4000, dead_time=3e-6, min_pw=5e-6, dp=off}
      mask prompts: fsw "Switching frequency [Hz]"; dead_time "Dead time [sec]"; min_pw "Minimum pulse width [sec]"; dp "Puls dropping"
      mask help: Implements a switching model for SV-PWM using C-SFunction
      mask init:
      | Tsw=1/fsw;
      | mpw=0.5*min_pw;
      mask Display: disp('Switching\nSVM\nC-SFun')
  Voltage Source Converter : Subsystem
      mask Type: Voltage Source Converter - star connected loads
      mask Description:
      | Implements a Voltage Source Converter (Rectifier or Inverter)
      | using switching functions.
      | - input S_ABC is          discret (0,1) => switching model.
      | - input S_ABC is continuous (0...1) =>   average model.
      mask Display: disp('VSC')

== system wt_blockset_v3/Transformations ==
  note: Transformations
  ABC->Mag&Phase : Subsystem
      mask Type: RMS&phase calculator
      mask Description: Calculate the RMS value and phase angle for a 3 phase input.
      mask Display: disp('')
  "DQ -> Complex" : Subsystem
      mask Type: DQ -> Complex
      mask Description: Transformation of dq variables into complex form
  "abc -> dq0" : Subsystem
      mask Description: Implements  ABC -> DQ  transformation
  "dq0 -> abc" : Subsystem
      mask Type: DQ -> ABC
      mask Description: Implements DQ -> ABC transformation
      mask Display: disp(' ')
  "phase -> line currents" : Subsystem
      mask Type: Transformation phase to line currents
      mask Description: Transformation of phase currents into line currents
      mask Display: disp('')
  phase->line voltages : Subsystem
      mask Type: Transformation phase to line voltages
      mask Description: Transformation of phase currents into line voltages
      mask Display: disp('')

== system wt_blockset_v3/Control/Active Stall Controller  ==
  wind : Inport  Port=1  LatchInput=off
  Ps : Inport  Port=2  LatchInput=off
  Pm : Inport  Port=3  LatchInput=off
  Enable : EnablePort  StatesWhenEnabling=reset
  Data Type Conversion : DataTypeConversion  SaturateOnIntegerOverflow=on  RndMeth=Zero
  Gain1 : Gain  Gain=1e-3  SaturateOnIntegerOverflow=on
  Gain2 : Gain  Gain=1*1e-3  SaturateOnIntegerOverflow=on
  MAF_wind : Subsystem  mask(Moving Average Filter){Tav=60, init=11.5}
      mask prompts: Tav "Averaging time interval [sec]"; init "Initial condition"
      mask help: Implements a Moving average filter in time domain
      mask Display: disp('Moving\nAverage')
  MAF_wind1 : Subsystem  mask(Moving Average Filter){Tav=5, init=1.8e6}
      mask prompts: Tav "Averaging time interval [sec]"; init "Initial condition"
      mask help: Implements a Moving average filter in time domain
      mask Display: disp('Moving\nAverage')
  Pitch System : Subsystem
  Power Controller : Subsystem
  Sample and Hold : Subsystem  TreatAsAtomicUnit=on  mask(Sample and Hold){trig=Rising edge, initCond=-1}
      mask prompts: trig "Trigger type:"; initCond "Initial condition:"
      mask help: Sample and hold input signal.
      mask init:
      | switch trig
      | case 1, s='rising';
      | case 2, s='falling';
      | case 3, s='either';
      | end
      | set_param([gcb '/Trigger'],'triggertype',s);
      mask Help: web(dspbhelp);
      mask StyleString: popup(Rising edge|Falling edge|Either edge),edit
      mask Display: disp('S/H')
  Saturation2 : Saturate  UpperLimit=-2  LowerLimit=-25
  Sum : Sum  Inputs=|+-  SaturateOnIntegerOverflow=on
  Switch : Switch  Threshold=0.5  SaturateOnIntegerOverflow=on
  control : Subsystem
  meas5 : Constant  Value=-Pallowed
  overpower  detection4 : RelationalOperator  Operator=>
  theta : Fcn  Expr=0.00068942619218*u(1)^3-0.04716431372377*u(1)^2+0.03911165958433*u(1)+2.45265812747683
  trigger : Subsystem
  pitch : Outport  InitialOutput=[-2.5]
  wires:
  Sum/1 -> overpower  detection4/2, Power Controller/1(error)  "error"
  Switch/1 -> Sample and Hold/1(In)
  Power Controller/1(pitch) -> Switch/3
  theta/1 -> Saturation2/1
  MAF_wind/1(Out) -> theta/1, control/1(av_wind)
  Pitch System/1(Out) -> pitch/1
  wind/1 -> MAF_wind/1(In)
  Ps/1 -> Gain1/1
  Pm/1 -> MAF_wind1/1(In)
  trigger/1(trigger) -> Sample and Hold/Trigger
  meas5/1 -> overpower  detection4/1
  overpower  detection4/1 -> Data Type Conversion/1
  Data Type Conversion/1 -> trigger/1(overpower)  "overpower"
  Saturation2/1 -> Switch/1  "optimum pitch"
  Sample and Hold/1(" ") -> Pitch System/1(In), Power Controller/2(aw)
  control/1(cs) -> Switch/2
  Gain1/1 -> Sum/1
  Gain2/1 -> Sum/2, control/2(error)
  MAF_wind1/1(Out) -> Gain2/1

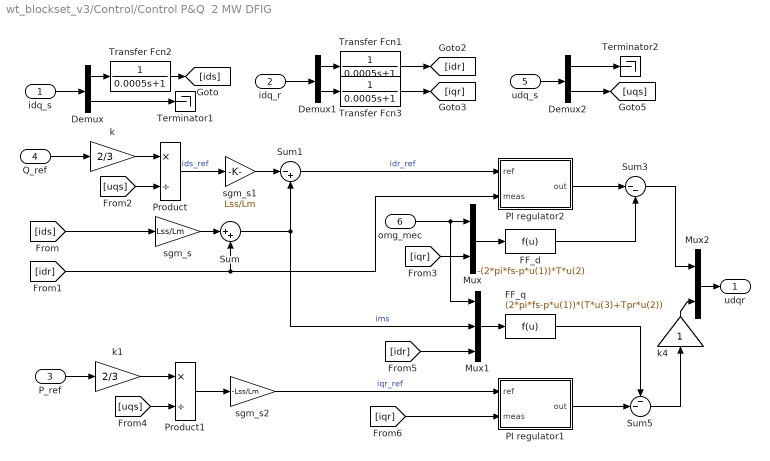
== system wt_blockset_v3/Control/Control P&Q  2 MW DFIG ==
  idq_s : Inport  Port=1  LatchInput=off
  idq_r : Inport  Port=2  LatchInput=off
  P_ref : Inport  Port=3  LatchInput=off
  Q_ref : Inport  Port=4  LatchInput=off
  udq_s : Inport  Port=5  LatchInput=off
  omg_mec : Inport  Port=6  LatchInput=off
  Demux : Demux  Outputs=2
  Demux1 : Demux  Outputs=2
  Demux2 : Demux  Outputs=2
  FF_d : Fcn  Expr=-(2*pi*fs-p*u(1))*T*u(2)
  FF_q : Fcn  Expr=(2*pi*fs-p*u(1))*(T*u(3)+Tpr*u(2))
  Mux : Mux  Inputs=2
  Mux1 : Mux  Inputs=3
  Mux2 : Mux  Inputs=2
  PI regulator1 : Subsystem  mask{K=0.002, Ti=0.04, ka=10, maxim=400, init_cond=0}
      mask prompts: K "Proportional Constant"; Ti "Integrate constant"; maxim "Limits"; init_cond "initial"
  PI regulator2 : Subsystem  mask{K=0.003, Ti=0.04, ka=10, maxim=400, init_cond=0}
      mask prompts: K "Proportional Constant"; Ti "Integrate constant"; maxim "Limits"; init_cond "initial"
  Product : Product  Inputs=*/  SaturateOnIntegerOverflow=on  InputSameDT=on
  Product1 : Product  Inputs=*/  SaturateOnIntegerOverflow=on  InputSameDT=on
  Sum : Sum  Inputs=|++  SaturateOnIntegerOverflow=on  InputSameDT=on
  Sum1 : Sum  Inputs=|-+  SaturateOnIntegerOverflow=on  InputSameDT=on
  Sum3 : Sum  Inputs=|--  SaturateOnIntegerOverflow=on  InputSameDT=on
  Sum5 : Sum  Inputs=--|  SaturateOnIntegerOverflow=on  InputSameDT=on
  Terminator1 : Terminator
  Terminator2 : Terminator
  Transfer Fcn1 : TransferFcn  Denominator=[0.0005 1]
  Transfer Fcn2 : TransferFcn  Denominator=[0.0005 1]
  Transfer Fcn3 : TransferFcn  Denominator=[0.0005 1]
  k : Gain  Gain=2/3  SaturateOnIntegerOverflow=on
  k1 : Gain  Gain=2/3  SaturateOnIntegerOverflow=on
  k4 : Gain  Orientation=up  SaturateOnIntegerOverflow=on
  sgm_s : Gain  Gain=Lss/Lm  SaturateOnIntegerOverflow=on
  sgm_s1 : Gain  Gain=Lss/Lm  SaturateOnIntegerOverflow=on
  sgm_s2 : Gain  Gain=-Lss/Lm  SaturateOnIntegerOverflow=on
  udqr : Outport
  wires:
  idq_s/1 -> Demux/1
  idq_r/1 -> Demux1/1
  Demux/1 -> Transfer Fcn2/1
  Demux/2 -> Terminator1/1
  Demux1/2 -> Transfer Fcn3/1
  [ids] -> sgm_s/1
  sgm_s/1 -> Sum/1
  [idr] -> Sum/2, PI regulator2/2(meas)
  udq_s/1 -> Demux2/1
  Demux2/1 -> Terminator2/1
  Demux2/2 -> [uqs]
  Q_ref/1 -> k/1
  k/1 -> Product/1
  [uqs] -> Product/2
  Product/1 -> sgm_s1/1  "ids_ref"
  Sum/1 -> Sum1/2, Mux1/2  "ims"
  PI regulator2/1(out) -> Sum3/1
  omg_mec/1 -> Mux/1, Mux1/1
  Mux/1 -> FF_d/1
  [iqr] -> Mux/2
  Sum3/1 -> Mux2/1
  P_ref/1 -> k1/1
  k1/1 -> Product1/1
  [uqs] -> Product1/2
  Product1/1 -> sgm_s2/1
  sgm_s2/1 -> PI regulator1/1(ref)  "iqr_ref"
  Mux1/1 -> FF_q/1
  PI regulator1/1(out) -> Sum5/2
  [idr] -> Mux1/3
  Sum5/1 -> k4/1
  Mux2/1 -> udqr/1
  sgm_s1/1 -> Sum1/1
  Sum1/1 -> PI regulator2/1(ref)  "idr_ref"
  FF_d/1 -> Sum3/2
  [iqr] -> PI regulator1/2(meas)
  Demux1/1 -> Transfer Fcn1/1
  Transfer Fcn2/1 -> [ids]
  Transfer Fcn1/1 -> [idr]
  Transfer Fcn3/1 -> [iqr]
  k4/1 -> Mux2/2
  FF_q/1 -> Sum5/1

== system wt_blockset_v3/Control/PI Controller anti wind-up ==
  error : Inport  Port=1  LatchInput=off
  1/T : Gain  Gain=1/Ti  SaturateOnIntegerOverflow=on
  Integrator : Integrator  InitialCondition=init_cond
  P1 : Gain  Gain=K  SaturateOnIntegerOverflow=on
  P2 : Gain  Orientation=left  Gain=ka  SaturateOnIntegerOverflow=on
  Saturation : Saturate  UpperLimit=maxim  LowerLimit=-maxim
  Sum1 : Sum  Inputs=|+-  SaturateOnIntegerOverflow=on  InputSameDT=on
  Sum2 : Sum  Inputs=++|  SaturateOnIntegerOverflow=on  InputSameDT=on
  Sum4 : Sum  Orientation=left  Inputs=+-|  SaturateOnIntegerOverflow=on  InputSameDT=on
  out : Outport  InitialOutput=0
  wires:
  Sum1/1 -> 1/T/1
  Integrator/1 -> Sum2/2
  1/T/1 -> Integrator/1
  error/1 -> P1/1
  P1/1 -> Sum1/1, Sum2/1
  P2/1 -> Sum1/2
  Sum2/1 -> Sum4/1, Saturation/1
  Sum4/1 -> P2/1
  Saturation/1 -> out/1, Sum4/2

== system wt_blockset_v3/Control/WT Controller 2 MW DFIG ==
  Pref_pu : Inport  Port=1  LatchInput=off
  Pmeas_pu : Inport  Port=2  LatchInput=off
  omg_meas : Inport  Port=3  LatchInput=off
  AAL : TransferFcn  Orientation=left  Denominator=[1e-4 1]
  Gain Scheduling : S-Function  Orientation=left  FunctionName=sfun_polyval  Parameters=coefs  mask(Polyval){coefs=[-2.0919e-008, 2.0362e-006, -8.1788e-005 1.7529e-003, -2.1671e-002, 1.5651e-001, -6.4415e-001, 1.4533e+000]}
      mask prompts: coefs "Polynomial coefficients:"
      mask help: Polynomial evaluation. Calculates P(u) given by the polynomial coefficient array P. P is sorted highest order to lowest order, the form accepted by MATLAB's polyval function.
      mask init:
      | if isempty(coefs)
      |   str = 'O(P) = ???';
      | else
      |   str = sprintf('O(P) = %d',length(coefs)-1);
      | end
      mask Display:
      | text(0.5,0.75, 'P(u)','horizontalAlignment','center')
      | text(0.5,0.25, str,'horizontalAlignment','center')
  Limit Power : Saturate  UpperLimit=0.6272  LowerLimit=0.0672
  Limit speed range : Saturate  UpperLimit=175.679  LowerLimit=83.77
  Optimum  speed : S-Function  FunctionName=sfun_polyval  Parameters=coefs  mask(Polyval){coefs=[-890.33 1543.7 -1074.6 467.9 53.548]}
      mask prompts: coefs "Polynomial coefficients:"
      mask help: Polynomial evaluation. Calculates P(u) given by the polynomial coefficient array P. P is sorted highest order to lowest order, the form accepted by MATLAB's polyval function.
      mask init:
      | if isempty(coefs)
      |   str = 'O(P) = ???';
      | else
      |   str = sprintf('O(P) = %d',length(coefs)-1);
      | end
      mask Display:
      | text(0.5,0.75, 'P(u)','horizontalAlignment','center')
      | text(0.5,0.25, str,'horizontalAlignment','center')
  Pitch System : Subsystem
  Power Controller : Subsystem  mask{K=Kp_power, Ti=Ti_power, ka=10, maxim=1, init_cond=0}
      mask prompts: K "Proportional Constant"; Ti "Integrate constant"; maxim "Limits"; init_cond "initial"
  Speed Controller : Subsystem  mask{K=Kp_speed, Ti=Ti_speed, ka=10, maxim=1000, init_cond=1}
      mask prompts: K "Proportional Constant"; Ti "Integrate constant"; maxim "Limits"; init_cond "initial"
  pitch : Outport
  Pref : Outport  Port=2
  wires:
  AAL/1 -> Gain Scheduling/1
  Gain Scheduling/1 -> Power Controller/3(Gain)
  Pref_pu/1 -> Power Controller/1(Ref), Limit Power/1
  Pmeas_pu/1 -> Power Controller/2(Meas)
  Power Controller/1(Out) -> Pitch System/1(In)
  Limit Power/1 -> Optimum  speed/1
  Optimum  speed/1 -> Limit speed range/1
  Limit speed range/1 -> Speed Controller/1(ref)
  Speed Controller/1(out) -> Pref/1
  omg_meas/1 -> Speed Controller/2(meas)
  Pitch System/1(Out) -> pitch/1, AAL/1

== system wt_blockset_v3/Control/control soft starter ==
  Enable : EnablePort
  Constant : Constant
  Constant1 : Constant  Value=110
  Gain1 : Gain  Gain=150  SaturateOnIntegerOverflow=on
  Integrator : Integrator
  Quantizer : Quantizer  QuantizationInterval=0.04  LinearizeAsGain=off
  Saturation : Saturate  UpperLimit=150  LowerLimit=70
  Sum : Sum  Inputs=|+-  SaturateOnIntegerOverflow=on  InputSameDT=on
  alpha : Outport
  wires:
  Saturation/1 -> alpha/1
  Quantizer/1 -> Gain1/1
  Constant/1 -> Integrator/1
  Integrator/1 -> Quantizer/1
  Gain1/1 -> Sum/2
  Constant1/1 -> Sum/1
  Sum/1 -> Saturation/1

== system wt_blockset_v3/Control/discrete PI Controller anti windup ==
  error : Inport  Port=1  LatchInput=off
  S-Function : S-Function  FunctionName=dscPI  Parameters=Kp, Ti, Ka, OutLim, Ts, InitCond
  out : Outport
  wires:
  error/1 -> S-Function/1
  S-Function/1 -> out/1

== system wt_blockset_v3/Electrical Machinery/C S-Function based  Models ==
  note: Electric Machines Dynamic Models
  note: C S-Function
      | based  Models
  note: DQ Reference frame
  note: ABC/abc Models
  note: Salient Pole
      | Synchronous Machine
  ABC/abc Squirrel Cage Induction Machine : Subsystem  mask(3-phase Induction Machine){Op_Mode=Generator, ConnType=D, stator=[3.67 9.2e-3], rotor=[2.32 12.29e-3], Lm=0.235, p=2, x0_init=[0 0 0 0 0]}
      mask prompts: Op_Mode "Operating mode"; ConnType "Connection type"; stator "Stator parameters [Rs (ohm), Lsgm_s (H)]"; rotor "Rotor parameters [Rr (ohm), Lsgm_r (H)]"; Lm "Magnetizing inductance [H]"; p "Number of poles pair"; x0_init "Initial conditions [iU iV iW iu iv iw theta]"
      mask help: This block implement the ABC dynamic model of the Induction Machine with constant parameters as an S-Function written in 'C' language
      mask init:
      | if ConnType==1,Type=1;else Type=-1;end
      | if Op_Mode==1, Kmode=1;else Kmode=-1;end
      mask StyleString: popup(Motor|Generator),popup(Y|D),edit,edit,edit,edit,edit
      mask Display: disp('ABC\nSC_IM')
  ABC/abc Wound Rotor Induction Machine : Subsystem  mask(3-phase Induction Machine){Op_Mode=Generator, ConnType=D, stator=[3.67 9.2e-3], rotor=[2.32 12.29e-3], Lm=0.235, p=2, x0_init=[0 0 0 0 0]}
      mask prompts: Op_Mode "Operating mode"; ConnType "Connection type"; stator "Stator parameters [Rs (ohm), Lsgm_s (H)]"; rotor "Rotor parameters [Rr (ohm), Lsgm_r (H)]"; Lm "Magnetizing inductance [H]"; p "Number of poles pair"; x0_init "Initial conditions [iU iV iW iu iv iw theta]"
      mask help: This block implement the ABC dynamic model of the Induction Machine with constant parameters as an S-Function written in 'C' language
      mask init:
      | if ConnType==1,Type=1;else Type=-1;end
      | if Op_Mode==1, Kmode=1;else Kmode=-1;end
      mask StyleString: popup(Motor|Generator),popup(Y|D),edit,edit,edit,edit,edit
      mask Display: disp('ABC\nSC_IM')
  DQ Salient-Pole Synchronous Machine : Subsystem  mask(Salient Pole Synchronous Machine){stator_winding=[2.34e-3 3.92e-4], field_winding=[5e-4 6.69246e-4], rotor_winding=[17.36e-3 5.22558e-4 16.75e-3 3.36082e-4], mag_ind=[2.3844e-3 1.1759e-3], p=32}
      mask prompts: stator_winding "Stator winding [Rs Lsgm_s]"; field_winding "Field winding [Rf Lsgm_f]"; rotor_winding "Rotor winding [Rrd Lsgm_rd Rrq Lsgm_rq]"; mag_ind "Magnetizing inductances [Lmd Lmq]"; p "Number of pole pairs"
      mask Display: disp('DQ\nSP_SP')
  DQ Squirrel Cage Induction Machine : Subsystem  mask(3-phase Induction Machine){stator=[3.67 9.2e-3], rotor=[2.32 12.29e-3], Lm=0.235, p=2, x0_init=[]}
      mask prompts: stator "Stator parameters [Rs (ohm), Lsgm_s (H)]"; rotor "Rotor parameters [Rr (ohm), Lsgm_r (H)]"; Lm "Magnetizing inductance [H]"; p "Number of poles pair"; x0_init "Initial conditions [ids iqs idr iqr theta]"
      mask help: This block implement the dynamic model of the Induction Machine with constant parameters as a S-Function written in 'C' language
      mask Display: disp('DQ\nSC_IM')
  DQ Wound Rotor Induction Machine : Subsystem  mask(3-phase Wound Rotor Induction Machine){stator=[0.01 95.5e-6], rotor=[0.01 95.5e-6], Lm=0.0955, p=2, x0_init=[]}
      mask prompts: stator "Stator parameters [Rs Lsgm_s] [ohms H]"; rotor "Rotor parameters [Rr Lsgm_r] [ohms H]"; Lm "Magnetizing inductance [H]"; p "Number of poles pair"; x0_init "Initial conditions [ids iqs idr' iqr' theta]"
      mask help: This block implement the dynamic model of the Wound Rotor Induction Machine with constant parameters as a S-Function written in 'C' language
      mask Display: disp('DQ\nWR_IM')
